simulink model "BugE_v0_40_MAS_loads"  (R2015b)
settings: Solver=FixedStepDiscrete  StartTime=0.0  StopTime=1980  FixedStep=sample_time  RelTol=1e-3
values from neighbouring files (symbols this model uses):
  AB_diode_dV = 0.9    [main_sync.m]
  air_density = 1.225    [main_sync.m]
  bus_charger_Pmax = 1000    [main_sync.m]
  bus_load_Pmax_abs = 250    [main_sync.m]
  capInitVolt = capVmax*sqrt(capInitSoC)    [main_sync.m]
  cyc_kph = [cyc_kph(:,1), cyc_kph(:,2)*speed_max_limit/speed_max]    [main_sync.m]
  cyc_repeat = 1    [main_sync.m]
  ess1_init_soc = 1    [main_sync.m]
  ess1_soh = 1    [main_sync.m]
  ess2_init_soc = 1    [main_sync.m]
  ess2_soh = 1    [main_sync.m]
  ess3_init_soc = 0.5    [main_sync.m]
  ess3_soh = 1    [main_sync.m]
  ess4_init_soc = 0.5    [main_sync.m]
  ess4_soh = 1    [main_sync.m]
  ess5_init_soc = 1    [main_sync.m]
  ess5_soh = 1    [main_sync.m]
  gear_ratio = 6    [main_sync.m]
  JADE_on = 1    [main_sync.m]
  loadpower = rawcsv(:,2)    [main_sync.m]
  loadtime = rawcsv(:,1)    [main_sync.m]
  lockSOCs = 0    [main_sync.m]
  max_brk_torque = 300    [main_sync.m]
  no_wheels = 3    [main_sync.m]
  period2 = max(loadtime)    [main_sync.m]
  PV_Pmax = 100    [main_sync.m]
  sample_time = 0.01    [main_sync.m]
  startup_seq_step_delay = 0.2    [main_sync.m]
  stop_option = 0    [main_sync.m]
  use_drive_cycle = 1    [main_sync.m]
  use_real_subs_loads = 1    [main_sync.m]
  vbus_max = 25    [main_sync.m]
  vbus_min = 17    [main_sync.m]
  vbus_safety_threshold = 2    [main_sync.m]
  vbus_threshold = 20    [main_sync.m]
  veh_CD = 0.35    [main_sync.m]
  veh_FA = 1.543    [main_sync.m]
  veh_gravity = 9.81*veh_mass    (= 1863.9)    [main_sync.m]
  veh_mass = 190    [main_sync.m]
  wh_1st_rrc = 0.02    [main_sync.m]
  wh_bearing_frc = 0.0015    [main_sync.m]
  wh_inertia = 0.0556    [main_sync.m]
  wh_radius = 0.508/2    (= 0.254)    [main_sync.m]
undefined symbols (not defined in the file or in its folder): capC, capR, cyc_acc, cyc_avg_time_samples, cyc_brk, cyc_grade, cyc_key, DCM_eff_factor_for_Vin, DCM_eff_for_Iout, DCM_Iout, DCM_Iout_max, DCM_Pin_noload, DCM_Pout_max, DCM_Vin, DCM_Vout, DiscIntNeverNeededParam, ess2_coulombic_eff, ess2_Ineg_max_SOC, ess2_Ineg_max_temp, ess2_Ipos_max_SOC, ess2_Ipos_max_temp, ess2_max_ah_cap, ess2_max_volts, ess2_min_volts, ess2_module_parallel, ess2_module_series, ess2_r_dis, ess2_soc, ess2_SOC_for_Ilimit, ess2_temp_for_Ilimit, ess2_temp_max, ess2_tmp, ess2_voc, ess3_coulombic_eff, ess3_max_ah_cap, ess3_module_parallel, ess3_module_series, ess3_r_dis, ess3_soc, ess3_tmp, ess3_voc, ess_coulombic_eff, ess_Ineg_max_SOC, ess_Ineg_max_temp, ess_Ipos_max_SOC, ess_Ipos_max_temp, ess_max_ah_cap, ess_max_volts, ess_min_volts, ess_module_parallel, ess_module_series, ess_nominal_volts, ess_r_dis, ess_soc, ess_SOC_for_Ilimit, ess_temp_for_Ilimit, ess_temp_max, ess_tmp, ess_voc, MC_eff1 ... (+17)
libraries: simulink x139, commfilt2 x1, simulink_extras x1
(part 1 of 7)
settings Model: Creator=gbucsan  LastModifiedBy=kcchu
settings DataIOCC: SaveFormat=Array
settings DebuggingCC: SolverPrmCheckMsg=warning  ParameterOverflowMsg=warning  AllowSymbolicDim=on
settings HardwareCC: ProdBitPerPointer=32  ProdLargestAtomicFloat=None  ProdIntDivRoundTo=Undefined  ProdEndianess=Unspecified  ProdWordSize=32  ProdHWDeviceType=32-bit Generic
settings ModelReferenceCC: ModelReferenceMinAlgLoopOccurrences=on
settings GRTTargetCC: GeneratePreprocessorConditionals=Disable all
settings ConfigComp: CovModelRefEnable=Off  CovSFcnEnable=off

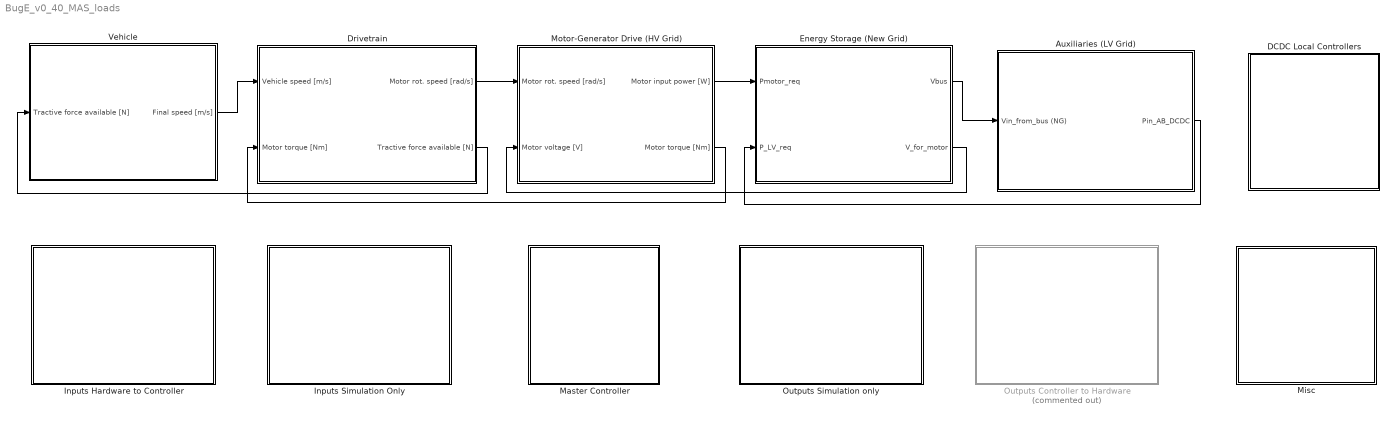
== system BugE_v0_40_MAS_loads ==
  Auxiliaries (LV Grid) : Subsystem
      mask Display: image('data\images\aux_systems2.png')
  DCDC Local Controllers : Subsystem
      mask Display: image('data\images\controller.png')
  Drivetrain : Subsystem
      mask Display: image('data\images\chain.jpg')
  Energy Storage (New Grid) : Subsystem
      mask Display: image('data\images\ess2.png')
  Inputs Hardware to Controller : Subsystem
      mask Display: image('data\images\in.png')
  Inputs Simulation Only : Subsystem
      mask Display: image('data\images\in.png')
  Master Controller : Subsystem
      mask Display: image('data\images\controller.png')
  Misc : Subsystem
      mask Display: image('data\images\debugger.png')
  Motor-Generator Drive (HV Grid) : Subsystem
      mask Display: image('data\images\motor.jpg')
  Outputs Controller to Hardware : Subsystem  Commented=on
      mask Display: image('data\images\out.png')
  Outputs Simulation only : Subsystem
      mask Display: image('data\images\out.png')
  Vehicle : Subsystem
      mask Display: image('data\images\bugev.png')
  wires:
  Vehicle/1(Final speed [m/s]) -> Drivetrain/1(Vehicle speed [m/s])
  Drivetrain/1(Motor rot. speed [rad/s]) -> Motor-Generator Drive (HV Grid)/1(Motor rot. speed [rad/s])
  Drivetrain/2(Tractive force available [N]) -> Vehicle/1(Tractive force available [N])
  Motor-Generator Drive (HV Grid)/2(Motor torque [Nm]) -> Drivetrain/2(Motor torque [Nm])
  Motor-Generator Drive (HV Grid)/1(Motor input power [W]) -> Energy Storage (New Grid)/1(Pmotor_req)
  Energy Storage (New Grid)/1("Vbus ") -> Auxiliaries (LV Grid)/1(Vin_from_bus (NG))
  Energy Storage (New Grid)/2(V_for_motor) -> Motor-Generator Drive (HV Grid)/2(Motor voltage [V])
  Auxiliaries (LV Grid)/1(Pin_AB_DCDC) -> Energy Storage (New Grid)/2(P_LV_req)

== system BugE_v0_40_MAS_loads/Auxiliaries (LV Grid) ==
  Vin_from_bus (NG) : Inport
  AB (w/ diode) : Subsystem
      mask Display: image('data\images\battery.jpg')
  AB DCDC : Subsystem
      mask Display: image('data\images\dcm.png')
  Auxiliary load (USB ports) : Subsystem
      mask Display: image('data\images\usb.jpg')
  Auxiliary load (lights) : Subsystem
      mask Display: image('data\images\auxiliaries.jpg')
  Constant : Constant  Value=0  SampleTime=sample_time
  ECU & sensors load : Subsystem
      mask Display: image('data\images\controller.png')
  P required on LV bus : Sum  Inputs=+++
  Switch1 : Switch  Criteria=u2 > Threshold
  Unit Delay1 : UnitDelay  InitialCondition=DCM_Pin_noload  SampleTime=sample_time
  Pin_AB_DCDC : Outport
  wires:
  Vin_from_bus (NG)/1 -> AB DCDC/1(Vin)
  AB DCDC/1(Pin_AB_DCDC (from new grid)) -> Unit Delay1/1
  Auxiliary load (lights)/1(power) -> P required on LV bus/1
  ECU & sensors load/1(power) -> P required on LV bus/2
  P required on LV bus/1 -> Switch1/1, AB DCDC/3(P_aux_req)
  [DDC] -> Switch1/2, AB DCDC/2(DCDC_enable)
  Switch1/1 -> AB (w/ diode)/1(Requested power [W])
  Unit Delay1/1 -> Pin_AB_DCDC/1
  Auxiliary load (USB ports)/1(power) -> P required on LV bus/3
  Constant/1 -> Switch1/3

== system BugE_v0_40_MAS_loads/DCDC Local Controllers ==
  Constant1 : Constant  Value=0
  Mux : Mux  Inputs=3
  Mux1 : Mux  Commented=on  Inputs=2
  Mux2 : Mux  Commented=on  Inputs=2
  Rate Transition3 : RateTransition
  Saturation Dynamic{,1..3} (4 alike) : simulink/Discontinuities/Saturation Dynamic  OutMin=[]  OutMax=[]  OutDataTypeStr=Inherit: Same as second input  OutDataType=fixdt(1, 16)  OutScaling=2^-10  DoSatur=off
  Scope : Scope  NumInputPorts=3
  To Workspace1 : ToWorkspace  VariableName=simout_Pmax_LD  SampleTime=1
  Unit Delay{1..4} (4 alike) : UnitDelay  SampleTime=-1
  flip sign : Gain  Gain=-1
  tag scope: PV_power_lim=global, ac_load_lim=global, autopilot_load_lim=global, charger_power_lim=global
  wires:
  [PV_power] -> Mux2/2, Saturation Dynamic/2  "pv"
  Constant1/1 -> Saturation Dynamic/3, Saturation Dynamic1/3, Saturation Dynamic3/3, Saturation Dynamic2/3
  [charger_power] -> Mux1/2, Saturation Dynamic1/2  "chg"
  [Chg_DCDC_command_value] -> Mux1/1, Saturation Dynamic1/1  "chg max"
  [Load_DCDC_command_value] -> flip sign/1  "load"
  flip sign/1 -> Rate Transition3/1, Mux/1, Saturation Dynamic3/1, Saturation Dynamic2/1  "load max"
  [autopilot_load] -> Mux/2, Saturation Dynamic2/2  "autopilot"
  Saturation Dynamic/1 -> Unit Delay1/1
  Saturation Dynamic1/1 -> Unit Delay2/1
  Saturation Dynamic2/1 -> Unit Delay3/1
  Unit Delay1/1 -> [PV_power_lim]
  Unit Delay2/1 -> [charger_power_lim]
  Unit Delay3/1 -> [autopilot_load_lim]
  [PV_DCDC_command_value] -> Mux2/1, Saturation Dynamic/1  "Pv max"
  Mux2/1 -> Scope/1
  Mux1/1 -> Scope/2
  Mux/1 -> Scope/3
  Saturation Dynamic3/1 -> Unit Delay4/1
  Unit Delay4/1 -> [ac_load_lim]
  [ac_load] -> Mux/3, Saturation Dynamic3/2  "A/C"
  Rate Transition3/1 -> To Workspace1/1

== system BugE_v0_40_MAS_loads/Drivetrain ==
  Vehicle speed [m/s] : Inport
  Motor torque [Nm] : Inport  Port=2
  "Brake_torque [Nm, abs]" : Gain  Gain=max_brk_torque
  Derivative : simulink/Discrete/Discrete Derivative  gainval=1.0  ICPrevScaledInput=0.0  InputProcessing=Inherited  OutMin=[]  OutMax=[]  OutDataType=fixdt(1, 16)  OutScaling=2^-10  DoSatur=off
  Energy Quantification : Subsystem
  Friction torque [Nm] : Product  Inputs=**
  Inertia torque [Nm] : Product  Inputs=**
  Speed [rad/s] : Product  Inputs=**
  Torque available at the wheel : Sum  Inputs=+---
  Torque available at the wheel sprocket from the motor [Nm] : Product
  Tractive force available : Product  Inputs=*/
  Wheel avg. rot. speed [rad/s] : Product  Inputs=/*
  "Wheel mom. of inertia [kg*m^2] " : Constant  Value=no_wheels*wh_inertia  SampleTime=sample_time
  gear ratio : Constant  Value=gear_ratio  SampleTime=sample_time
  wheel bearing viscous friction coeff.[Nm/(rad/s)] : Constant  Value=no_wheels*wh_bearing_frc  SampleTime=sample_time
  wheel radius [m] : Constant  Value=wh_radius  SampleTime=sample_time
  Motor rot. speed [rad/s] : Outport
  Tractive force available [N] : Outport  Port=2
  wires:
  Derivative/1 -> Inertia torque [Nm]/1
  wheel radius [m]/1 -> Tractive force available/2, Wheel avg. rot. speed [rad/s]/1
  Motor torque [Nm]/1 -> Torque available at the wheel sprocket from the motor [Nm]/2
  "Wheel mom. of inertia [kg*m^2] "/1 -> Inertia torque [Nm]/2
  wheel bearing viscous friction coeff.[Nm/(rad/s)]/1 -> Friction torque [Nm]/2
  Torque available at the wheel sprocket from the motor [Nm]/1 -> Torque available at the wheel/1
  Speed [rad/s]/1 -> Motor rot. speed [rad/s]/1
  Vehicle speed [m/s]/1 -> Wheel avg. rot. speed [rad/s]/2
  Tractive force available/1 -> Tractive force available [N]/1
  Torque available at the wheel/1 -> Tractive force available/1
  gear ratio/1 -> Speed [rad/s]/1, Torque available at the wheel sprocket from the motor [Nm]/1
  Inertia torque [Nm]/1 -> Torque available at the wheel/3, Energy Quantification/4(In4)
  Friction torque [Nm]/1 -> Energy Quantification/3(In3), Torque available at the wheel/2
  Wheel avg. rot. speed [rad/s]/1 -> Derivative/1, Friction torque [Nm]/1, Energy Quantification/2(In2), Speed [rad/s]/2
  "Brake_torque [Nm, abs]"/1 -> Energy Quantification/1(In1), Torque available at the wheel/4
  [brake] -> "Brake_torque [Nm, abs]"/1

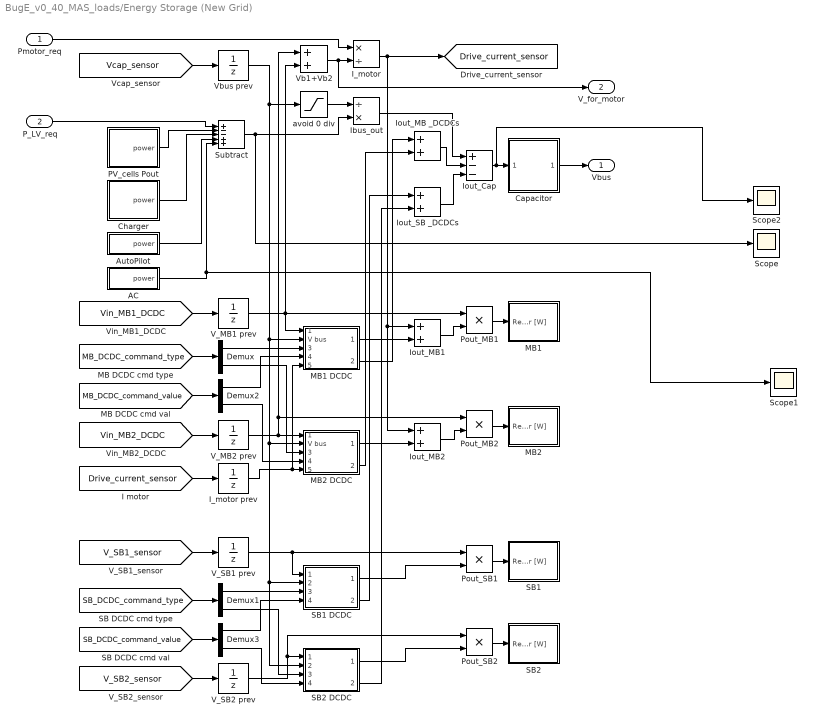
== system BugE_v0_40_MAS_loads/Energy Storage (New Grid) ==
  Pmotor_req : Inport
  P_LV_req : Inport  Port=2
  AC : Subsystem
  AutoPilot : Subsystem
  Capacitor : Subsystem
      mask Display: image('data\images\dlcap.jpg')
  Charger : Subsystem
      mask Display: image('data\images\v2g.jpg')
  Demux{,1..3} (4 alike) : Demux  Outputs=2
  I_motor : Product  Inputs=*/
  I_motor prev : UnitDelay  SampleTime=sample_time
  Ibus_out : Product  Inputs=/*
  Iout_Cap : Sum  Inputs=+--
  Iout_MB _DCDCs : Sum
  Iout_MB1 : Sum
  Iout_MB2 : Sum
  Iout_SB _DCDCs : Sum
  MB1 : Subsystem
      mask Display: image('data\images\battery.jpg')
  MB1 DCDC : Subsystem
      mask Display: image('data\images\dab.jpg')
  MB2 : Subsystem
      mask Display: image('data\images\battery.jpg')
  MB2 DCDC : Subsystem
      mask Display: image('data\images\dab.jpg')
  PV_cells Pout : Subsystem
      mask Display: image('data\images\pv.jpg')
  Pout_MB1 : Product
  Pout_MB2 : Product
  Pout_SB1 : Product
  Pout_SB2 : Product
  SB1 : Subsystem
      mask Display: image('data\images\battery.jpg')
  SB1 DCDC : Subsystem
      mask Display: image('data\images\dab.jpg')
  SB2 : Subsystem
      mask Display: image('data\images\battery.jpg')
  SB2 DCDC : Subsystem
      mask Display: image('data\images\dab.jpg')
  Scope : Scope
  Scope1 : Scope
  Scope2 : Scope
  Subtract : Sum  Inputs=+--++
  V_MB1 prev : UnitDelay  InitialCondition=ess_module_series*ess_max_volts  SampleTime=-1
  V_MB2 prev : UnitDelay  InitialCondition=ess_module_series*ess_max_volts  SampleTime=-1
  V_SB1 prev : UnitDelay  InitialCondition=ess2_module_series*ess2_max_volts  SampleTime=-1
  V_SB2 prev : UnitDelay  InitialCondition=ess2_module_series*ess2_max_volts  SampleTime=-1
  Vb1+Vb2 : Sum
  Vbus prev : UnitDelay  InitialCondition=capInitVolt  SampleTime=-1
  avoid 0 div : Saturate  UpperLimit=inf  LowerLimit=eps
  "Vbus " : Outport
  V_for_motor : Outport  Port=2
  tag scope: Drive_current_sensor=global
  wires:
  Pmotor_req/1 -> I_motor/1
  Vb1+Vb2/1 -> V_for_motor/1, I_motor/2
  MB1 DCDC/1(DAB_I_in) -> Iout_MB1/2
  MB2 DCDC/1(DAB_I_in) -> Iout_MB2/2
  Iout_MB2/1 -> Pout_MB2/2
  Iout_MB1/1 -> Pout_MB1/2
  Pout_MB1/1 -> MB1/1(Requested power [W])
  Pout_MB2/1 -> MB2/1(Requested power [W])
  MB2 DCDC/2(DAB_I_out) -> Iout_MB _DCDCs/2
  Ibus_out/1 -> Iout_Cap/1
  Subtract/1 -> Scope/1, Ibus_out/2
  Capacitor/1(Vbus) -> "Vbus "/1
  [Vin_MB1_DCDC] -> V_MB1 prev/1
  V_MB1 prev/1 -> MB1 DCDC/1(V batt), Vb1+Vb2/2, Pout_MB1/1
  [Vin_MB2_DCDC] -> V_MB2 prev/1
  V_MB2 prev/1 -> MB2 DCDC/1(V batt), Vb1+Vb2/1, Pout_MB2/1
  [Vcap_sensor] -> Vbus prev/1
  Iout_MB _DCDCs/1 -> Iout_Cap/2
  [V_SB1_sensor] -> V_SB1 prev/1
  V_SB1 prev/1 -> SB1 DCDC/1(V batt), Pout_SB1/1
  Vbus prev/1 -> MB2 DCDC/2(V bus), SB2 DCDC/2(V bus), SB1 DCDC/2(V bus), MB1 DCDC/2(V bus), avoid 0 div/1
  [V_SB2_sensor] -> V_SB2 prev/1
  V_SB2 prev/1 -> SB2 DCDC/1(V batt), Pout_SB2/1
  SB1 DCDC/1(DAB_I_in) -> Pout_SB1/2
  SB2 DCDC/1(DAB_I_in) -> Pout_SB2/2
  Pout_SB1/1 -> SB1/1(Requested power [W])
  Pout_SB2/1 -> SB2/1(Requested power [W])
  SB2 DCDC/2(DAB_I_out) -> Iout_SB _DCDCs/2
  SB1 DCDC/2(DAB_I_out) -> Iout_SB _DCDCs/1
  Iout_SB _DCDCs/1 -> Iout_Cap/3
  P_LV_req/1 -> Subtract/1
  PV_cells Pout/1(power) -> Subtract/2
  Charger/1(power) -> Subtract/3
  AutoPilot/1(power) -> Subtract/4
  avoid 0 div/1 -> Ibus_out/1
  Demux/1 -> MB1 DCDC/3("cmd type 0 P, 1 V ")
  [MB_DCDC_command_type] -> Demux/1
  [MB_DCDC_command_value] -> Demux2/1
  Demux2/1 -> MB1 DCDC/4(cmd value)
  [Drive_current_sensor] -> I_motor prev/1
  Demux/2 -> MB2 DCDC/3("cmd type 0 P, 1 V ")
  Demux2/2 -> MB2 DCDC/4(cmd value)
  I_motor prev/1 -> MB2 DCDC/5(I motor), MB1 DCDC/5(I motor)
  [SB_DCDC_command_type] -> Demux1/1
  [SB_DCDC_command_value] -> Demux3/1
  Demux1/1 -> SB1 DCDC/3("cmd type 0 P, 1 V ")
  Demux1/2 -> SB2 DCDC/3("cmd type 0 P, 1 V ")
  Demux3/1 -> SB1 DCDC/4(cmd value)
  Demux3/2 -> SB2 DCDC/4(cmd value)
  MB1 DCDC/2(DAB_I_out) -> Iout_MB _DCDCs/1
  I_motor/1 -> [Drive_current_sensor], Iout_MB1/1, Iout_MB2/1
  AC/1(power) -> Subtract/5, Scope1/1
  Iout_Cap/1 -> Scope2/1, Capacitor/1(Iout_RC)

== system BugE_v0_40_MAS_loads/Inputs Hardware to Controller ==
  Device detection & identification : Subsystem
  Sensors and readings : Subsystem
  User Inputs : Subsystem

== system BugE_v0_40_MAS_loads/Inputs Simulation Only ==
  AC load : Subsystem
  Autopilot load : Subsystem
  Auxiliaries power : Subsystem
  Charger power : Subsystem
  Clock1 : Clock
  Command Cycles : Subsystem
      mask Display: image('data\images\commands.png')
  PV power : Subsystem
  Standby load : Subsystem
  USB power : Subsystem
  dt : Constant  Value=sample_time  SampleTime=sample_time
  ess1_init_soc : Constant  Value=ess1_init_soc  SampleTime=sample_time
  ess2_init_soc : Constant  Value=ess2_init_soc  SampleTime=sample_time
  ess5_init_soc : Constant  Value=ess5_init_soc  SampleTime=sample_time
  repeat1 : Constant  Value=cyc_repeat  SampleTime=sample_time
  zero : Constant  Value=0  SampleTime=sample_time
  tag scope: AB_SOCinit=global, MB1_SOCinit=global, MB1_lower_SOH=global, MB2_SOCinit=global, PV_power=global, USB_load=global, ac_load=global, autopilot_load=global, aux_load=global, brake=global, charger_power=global, dt=global, endcycle_stopsim=global, grade=global, standby_load=global
  wires:
  zero/1 -> [MB1_lower_SOH]
  Standby load/1(Out1) -> [standby_load]
  Auxiliaries power/1(Out1) -> [aux_load]
  Autopilot load/1(Out1) -> [autopilot_load]
  Charger power/1(Out1) -> [charger_power]
  PV power/1(Out1) -> [PV_power]
  ess1_init_soc/1 -> [MB1_SOCinit]
  ess2_init_soc/1 -> [MB2_SOCinit]
  ess5_init_soc/1 -> [AB_SOCinit]
  Clock1/1 -> Command Cycles/2(Time)
  repeat1/1 -> Command Cycles/1(repeat)
  Command Cycles/2(endcycle_stopsim) -> [endcycle_stopsim]
  Command Cycles/3(grade) -> [grade]
  dt/1 -> [dt]
  Command Cycles/1(acc_brk_out) -> [brake]
  USB power/1(Out1) -> [USB_load]
  AC load/1(Out1) -> [ac_load]

== system BugE_v0_40_MAS_loads/Master Controller ==
  DCDC Calculators : Subsystem
  Detection : Subsystem
  Motor Controller : Subsystem
  Operating Mode Controller : Subsystem
  Secondary Objectives : Subsystem
  Signal Buffer : Subsystem
  System Health : Subsystem

== system BugE_v0_40_MAS_loads/Misc ==
  Data logging : Subsystem
  Debugging : Subsystem
  Energy Calculations : Subsystem
      mask Display: image('data\images\pie.png')
  STOP Sim : Subsystem

== system BugE_v0_40_MAS_loads/Motor-Generator Drive (HV Grid) ==
  Motor rot. speed [rad/s] : Inport
  Motor voltage [V] : Inport  Port=2
  Constant : Constant  Value=0  SampleTime=sample_time
  Current limiter : Subsystem
  Delay : Delay  DelayLength=1  SampleTime=sample_time
  Discrete Derivative : simulink/Discrete/Discrete Derivative  gainval=1.0  ICPrevScaledInput=0.0  InputProcessing=Inherited  OutMin=[]  OutMax=[]  OutDataType=fixdt(1, 16)  OutScaling=2^-10  DoSatur=off
  Efficiency map : Lookup_n-D  BreakpointsForDimension1=mc_map_spd*mc_spd_scale  BreakpointsForDimension2=mc_map_trq*mc_trq_scale  Table=mc_inpwr_map*mc_spd_scale*mc_trq_scale  InternalRulePriority=Speed  SaturateOnIntegerOverflow=on  InputSameDT=on
  Energy Quantification : Subsystem
  Gain : Gain  Gain=-1
  Inertia trq : Gain  Gain=mc_inertia
  Switch_Motor on/off : Switch  Criteria=u2 > Threshold
  Switch_Motor on/off1 : Switch  Criteria=u2 > Threshold
  Torque limiter : Subsystem
  Total torque output [Nm] : Sum  Inputs=+-
  Unit Delay prevent timing errors : UnitDelay  SampleTime=sample_time
  Motor input power [W] : Outport
  Motor torque [Nm] : Outport  Port=2
  wires:
  Efficiency map/1 -> Current limiter/1(Input power [W])
  Switch_Motor on/off/1 -> Energy Quantification/1(Pin), Motor input power [W]/1
  Torque limiter/1(Limited req. trq) -> Current limiter/3(Req. torque), Efficiency map/2
  Inertia trq/1 -> Energy Quantification/4(inertia torque), Gain/1, Total torque output [Nm]/2, Torque limiter/2(Inertia torque [Nm])
  Discrete Derivative/1 -> Inertia trq/1
  Motor voltage [V]/1 -> Current limiter/2(Voltage [V])
  Current limiter/1(Limited input power) -> Switch_Motor on/off/1
  Constant/1 -> Switch_Motor on/off/3
  [RLY_DRV] -> Unit Delay prevent timing errors/1
  Switch_Motor on/off1/1 -> Energy Quantification/3(torque out), Motor torque [Nm]/1
  Motor rot. speed [rad/s]/1 -> Discrete Derivative/1, Efficiency map/1, Energy Quantification/2(speed), Torque limiter/1(Speed [rad/s])
  Current limiter/2(Limited torque) -> Total torque output [Nm]/1
  Total torque output [Nm]/1 -> Switch_Motor on/off1/1
  Gain/1 -> Switch_Motor on/off1/3
  [throttle_adjusted] -> Delay/1
  Delay/1 -> Torque limiter/3(Requested throttle [0-1])
  Unit Delay prevent timing errors/1 -> Switch_Motor on/off/2, Switch_Motor on/off1/2

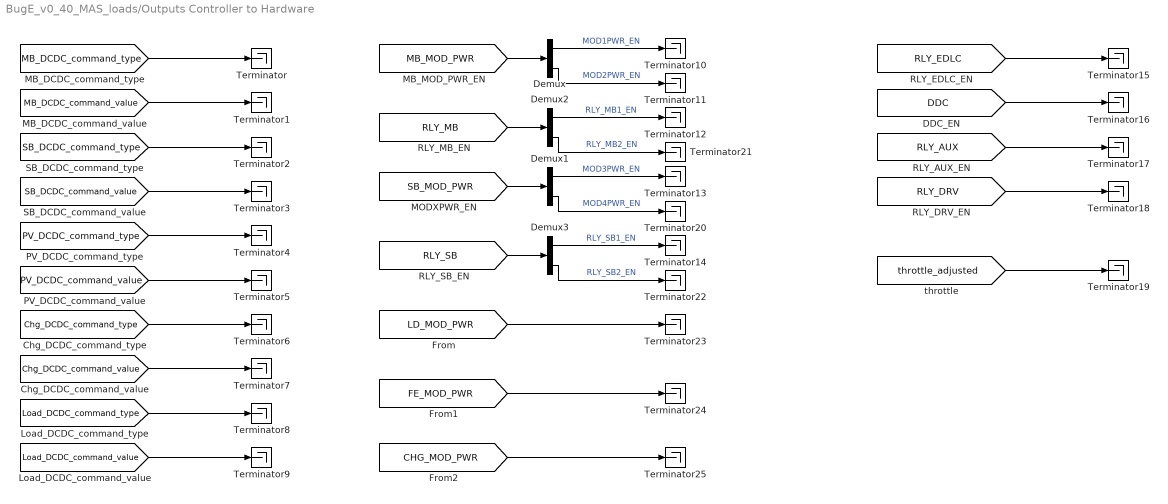
== system BugE_v0_40_MAS_loads/Outputs Controller to Hardware ==
  Demux{,1..3} (4 alike) : Demux  Outputs=2
  Terminator{,1..25} (26 alike) : Terminator
  wires:
  [MB_DCDC_command_type] -> Terminator/1
  [MB_DCDC_command_value] -> Terminator1/1
  [SB_DCDC_command_type] -> Terminator2/1
  [SB_DCDC_command_value] -> Terminator3/1
  [PV_DCDC_command_type] -> Terminator4/1
  [PV_DCDC_command_value] -> Terminator5/1
  [Chg_DCDC_command_type] -> Terminator6/1
  [Chg_DCDC_command_value] -> Terminator7/1
  [Load_DCDC_command_type] -> Terminator8/1
  [Load_DCDC_command_value] -> Terminator9/1
  Demux/1 -> Terminator10/1  "MOD1PWR_EN"
  Demux/2 -> Terminator11/1  "MOD2PWR_EN"
  [RLY_EDLC] -> Terminator15/1
  [DDC] -> Terminator16/1
  [RLY_AUX] -> Terminator17/1
  [RLY_DRV] -> Terminator18/1
  [throttle_adjusted] -> Terminator19/1
  [MB_MOD_PWR] -> Demux/1
  Demux1/1 -> Terminator13/1  "MOD3PWR_EN"
  Demux1/2 -> Terminator20/1  "MOD4PWR_EN"
  [SB_MOD_PWR] -> Demux1/1
  Demux2/1 -> Terminator12/1  "RLY_MB1_EN"
  Demux2/2 -> Terminator21/1  "RLY_MB2_EN"
  [RLY_MB] -> Demux2/1
  Demux3/1 -> Terminator14/1  "RLY_SB1_EN"
  Demux3/2 -> Terminator22/1  "RLY_SB2_EN"
  [RLY_SB] -> Demux3/1
  [LD_MOD_PWR] -> Terminator23/1
  [FE_MOD_PWR] -> Terminator24/1
  [CHG_MOD_PWR] -> Terminator25/1

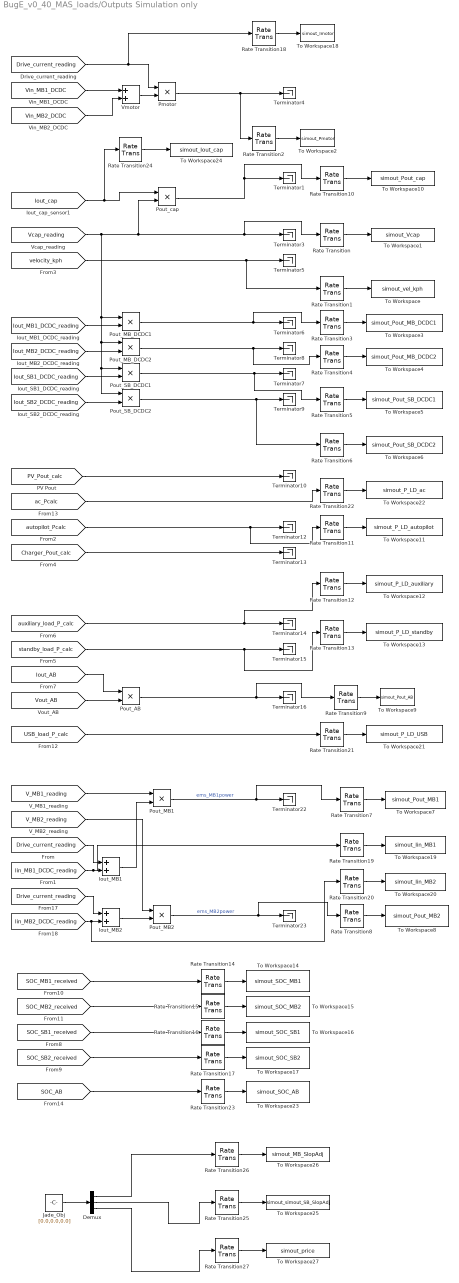
== system BugE_v0_40_MAS_loads/Outputs Simulation only ==
  Demux : Demux  Outputs=3
  Iout_MB1 : Sum
  Iout_MB2 : Sum
  Jade_Obj : Constant  Value=[0.0,0.0,0.0]  SampleTime=sample_time
  Pmotor : Product
  Pout_AB : Product
  Pout_MB1 : Product
  Pout_MB2 : Product
  Pout_MB_DCDC1 : Product
  Pout_MB_DCDC2 : Product
  Pout_SB_DCDC1 : Product
  Pout_SB_DCDC2 : Product
  Pout_cap : Product
  Rate Transition{,1..27} (28 alike) : RateTransition
  Terminator{1,3..10,12..16,22..23} (16 alike) : Terminator
  To Workspace : ToWorkspace  VariableName=simout_vel_kph  SampleTime=1
  To Workspace1 : ToWorkspace  VariableName=simout_Vcap  SampleTime=1
      settings: MaxDataPoints=Inf
  To Workspace10 : ToWorkspace  VariableName=simout_Pout_cap  SampleTime=1
      settings: MaxDataPoints=Inf
  To Workspace11 : ToWorkspace  VariableName=simout_P_LD_autopilot  SampleTime=1
  To Workspace12 : ToWorkspace  VariableName=simout_P_LD_auxiliary  SampleTime=1
  To Workspace13 : ToWorkspace  VariableName=simout_P_LD_standby  SampleTime=1
  To Workspace14 : ToWorkspace  VariableName=simout_SOC_MB1  SampleTime=1
  To Workspace15 : ToWorkspace  VariableName=simout_SOC_MB2  SampleTime=1
  To Workspace16 : ToWorkspace  VariableName=simout_SOC_SB1  SampleTime=1
  To Workspace17 : ToWorkspace  VariableName=simout_SOC_SB2  SampleTime=1
  To Workspace18 : ToWorkspace  VariableName=simout_Imotor  SampleTime=1
  To Workspace19 : ToWorkspace  VariableName=simout_Iin_MB1  SampleTime=1
  To Workspace2 : ToWorkspace  VariableName=simout_Pmotor  SampleTime=1
  To Workspace20 : ToWorkspace  VariableName=simout_Iin_MB2  SampleTime=1
  To Workspace21 : ToWorkspace  VariableName=simout_P_LD_USB  SampleTime=1
  To Workspace22 : ToWorkspace  VariableName=simout_P_LD_ac  SampleTime=1
  To Workspace23 : ToWorkspace  VariableName=simout_SOC_AB  SampleTime=1
  To Workspace24 : ToWorkspace  VariableName=simout_Iout_cap  SampleTime=1
      settings: MaxDataPoints=Inf
  To Workspace25 : ToWorkspace  VariableName=simout_simout_SB_SlopAdj  SampleTime=1
      settings: MaxDataPoints=Inf
  To Workspace26 : ToWorkspace  VariableName=simout_MB_SlopAdj  SampleTime=1
      settings: MaxDataPoints=Inf
  To Workspace27 : ToWorkspace  VariableName=simout_price  SampleTime=1
      settings: MaxDataPoints=Inf
  To Workspace3 : ToWorkspace  VariableName=simout_Pout_MB_DCDC1  SampleTime=1
  To Workspace4 : ToWorkspace  VariableName=simout_Pout_MB_DCDC2  SampleTime=1
  To Workspace5 : ToWorkspace  VariableName=simout_Pout_SB_DCDC1  SampleTime=1
  To Workspace6 : ToWorkspace  VariableName=simout_Pout_SB_DCDC2  SampleTime=1
  To Workspace7 : ToWorkspace  VariableName=simout_Pout_MB1  SampleTime=1
  To Workspace8 : ToWorkspace  VariableName=simout_Pout_MB2  SampleTime=1
  To Workspace9 : ToWorkspace  VariableName=simout_Pout_AB  SampleTime=1
  Vmotor : Sum
  wires:
  Vmotor/1 -> Pmotor/2
  [Vin_MB2_DCDC] -> Vmotor/2
  [Drive_current_reading] -> Rate Transition18/1, Pmotor/1
  Pmotor/1 -> Rate Transition2/1, Terminator4/1
  [Vin_MB1_DCDC] -> Vmotor/1
  [Vcap_reading] -> Pout_cap/2, Rate Transition/1, Terminator3/1, Pout_SB_DCDC2/1, Pout_SB_DCDC1/1, Pout_MB_DCDC2/1, Pout_MB_DCDC1/1
  [velocity_kph] -> Rate Transition1/1, Terminator5/1
  [Iout_MB1_DCDC_reading] -> Pout_MB_DCDC1/2
  [Iout_MB2_DCDC_reading] -> Pout_MB_DCDC2/2
  [Iout_SB1_DCDC_reading] -> Pout_SB_DCDC1/2
  [Iout_SB2_DCDC_reading] -> Pout_SB_DCDC2/2
  Pout_MB_DCDC1/1 -> Rate Transition3/1, Terminator6/1
  Pout_MB_DCDC2/1 -> Rate Transition4/1, Terminator8/1
  Pout_SB_DCDC1/1 -> Rate Transition5/1, Terminator7/1
  Pout_SB_DCDC2/1 -> Rate Transition6/1, Terminator9/1
  [PV_Pout_calc] -> Terminator10/1
  [autopilot_Pcalc] -> Rate Transition11/1, Terminator12/1
  [Charger_Pout_calc] -> Terminator13/1
  [Vout_AB] -> Pout_AB/2
  [Iout_AB] -> Pout_AB/1
  Pout_AB/1 -> Rate Transition9/1, Terminator16/1
  Iout_MB2/1 -> Pout_MB2/2
  [V_MB2_reading] -> Pout_MB2/1
  [V_MB1_reading] -> Pout_MB1/1
  Iout_MB1/1 -> Pout_MB1/2
  Pout_MB1/1 -> Rate Transition7/1, Terminator22/1  "ems_MB1power"
  Pout_MB2/1 -> Rate Transition8/1, Terminator23/1  "ems_MB2power"
  [Drive_current_reading] -> Iout_MB1/1
  [Iin_MB1_DCDC_reading] -> Rate Transition19/1, Iout_MB1/2
  [Drive_current_reading] -> Iout_MB2/1
  [Iin_MB2_DCDC_reading] -> Rate Transition20/1, Iout_MB2/2
  Rate Transition/1 -> To Workspace1/1
  Rate Transition1/1 -> To Workspace/1
  Rate Transition2/1 -> To Workspace2/1
  Rate Transition3/1 -> To Workspace3/1
  Rate Transition4/1 -> To Workspace4/1
  Rate Transition5/1 -> To Workspace5/1
  Rate Transition6/1 -> To Workspace6/1
  Rate Transition7/1 -> To Workspace7/1
  Rate Transition8/1 -> To Workspace8/1
  Rate Transition9/1 -> To Workspace9/1
  [Iout_cap] -> Rate Transition24/1, Pout_cap/1
  Pout_cap/1 -> Rate Transition10/1, Terminator1/1
  Rate Transition10/1 -> To Workspace10/1
  Rate Transition11/1 -> To Workspace11/1
  [auxiliary_load_P_calc] -> Rate Transition12/1, Terminator14/1
  Rate Transition12/1 -> To Workspace12/1
  [standby_load_P_calc] -> Rate Transition13/1, Terminator15/1
  Rate Transition13/1 -> To Workspace13/1
  Rate Transition14/1 -> To Workspace14/1
  [SOC_MB1_received] -> Rate Transition14/1
  Rate Transition15/1 -> To Workspace15/1
  [SOC_MB2_received] -> Rate Transition15/1
  Rate Transition16/1 -> To Workspace16/1
  [SOC_SB1_received] -> Rate Transition16/1
  Rate Transition17/1 -> To Workspace17/1
  [SOC_SB2_received] -> Rate Transition17/1
  Rate Transition18/1 -> To Workspace18/1
  Rate Transition19/1 -> To Workspace19/1
  Rate Transition20/1 -> To Workspace20/1
  [USB_load_P_calc] -> Rate Transition21/1
  Rate Transition21/1 -> To Workspace21/1
  Rate Transition22/1 -> To Workspace22/1
  [ac_Pcalc] -> Rate Transition22/1
  Rate Transition23/1 -> To Workspace23/1
  [SOC_AB] -> Rate Transition23/1
  Rate Transition24/1 -> To Workspace24/1
  Jade_Obj/1 -> Demux/1
  Demux/2 -> Rate Transition25/1
  Rate Transition25/1 -> To Workspace25/1
  Demux/1 -> Rate Transition26/1
  Rate Transition26/1 -> To Workspace26/1
  Demux/3 -> Rate Transition27/1
  Rate Transition27/1 -> To Workspace27/1

== system BugE_v0_40_MAS_loads/Vehicle ==
  Tractive force available [N] : Inport
  Achievable vehicle speed : Subsystem
  Unit Delay : UnitDelay  SampleTime=-1
  "m/s -> km/h" : Gain  Gain=3.6
  Final speed [m/s] : Outport
  tag scope: velocity_kph=global
  wires:
  Tractive force available [N]/1 -> Achievable vehicle speed/2(Available avg. tractive force [N])
  Achievable vehicle speed/1(Vehicle speed at the end of time step [m/s]) -> Unit Delay/1, "m/s -> km/h"/1
  "m/s -> km/h"/1 -> [velocity_kph]
  Unit Delay/1 -> Achievable vehicle speed/1(Vehicle speed at the beginning of the time step [m/s]), Final speed [m/s]/1

== system BugE_v0_40_MAS_loads/Auxiliaries (LV Grid)/AB (w// diode) ==
  Requested power [W] : Inport
  AB_diode_dV : Constant  Value=AB_diode_dV  SampleTime=sample_time
  Calculate SOC : Subsystem
  Compute current (nolimit) : Subsystem
  Constant : Constant  Value=25  SampleTime=sample_time
  Energy Quantification : Subsystem
  "Pack Voc, R" : Subsystem
  Scope : Scope
  tag scope: Iout_AB=global, SOC_AB=global, Vout_AB=global
  wires:
  Requested power [W]/1 -> "Pack Voc, R"/3(Req. power [W]), Compute current (nolimit)/3(Output power [W])
  "Pack Voc, R"/1(Pack Voc [V]) -> Compute current (nolimit)/1(Voc [V])
  Constant/1 -> Calculate SOC/1(Temp [C]), "Pack Voc, R"/1(Temp [degC])
  [SOC_AB] -> "Pack Voc, R"/2(SOC_prev)
  "Pack Voc, R"/2(Pack R [Ohm]) -> Energy Quantification/3(R), Compute current (nolimit)/2(Rint [Ohm])
  Compute current (nolimit)/1(I [A]) -> Calculate SOC/2(I [A]), [Iout_AB], Energy Quantification/2(Iout)
  AB_diode_dV/1 -> Compute current (nolimit)/4(diode_dV [V]), Energy Quantification/4(diode_dV [V])
  Compute current (nolimit)/2(V_out [V]) -> Energy Quantification/1(Vout), [Vout_AB]
  Calculate SOC/1(SOC) -> Scope/1, [SOC_AB]

== system BugE_v0_40_MAS_loads/Auxiliaries (LV Grid)/AB DCDC ==
  Vin : Inport
  DCDC_enable : Inport  Port=2
  P_aux_req : Inport  Port=3
  >0 avoid 0 div : Saturate  UpperLimit=inf  LowerLimit=eps
  Comp 0 : simulink/Logic and Bit Operations/Compare To Zero  relop===  OutDataTypeStr=boolean
  Constant : Constant  Value=0  SampleTime=sample_time
  DCM: Iout->eff : Lookup_n-D  NumberOfTableDimensions=1  BreakpointsForDimension1=DCM_Iout(:)  Table=DCM_eff_for_Iout(:)  InterpMethod=Cubic spline  ExtrapMethod=Clip  InternalRulePriority=Speed  RndMeth=Simplest  InputSameDT=on
  Energy Quantification : Subsystem
  Iin : Product  Inputs=*/
  Imax : Constant  Value=DCM_Iout_max  SampleTime=sample_time
  Iout : Product  Inputs=*/
  Iout_AB_DCDC_sensor : Goto  Commented=on  GotoTag=Iout_AB_DCDC_sensor  TagVisibility=global
  Min : MinMax  Inputs=2
  P=0 for shutdown : Switch  Criteria=u2 > Threshold
  P_noload : Constant  Value=DCM_Pin_noload  SampleTime=sample_time
  Pin_init : Product  Inputs=*/
  Pin_init1 : Product  Inputs=*/
  Pmax : MinMax  Inputs=2
  Pmax_calc : Product
  Pmax_given : Constant  Value=DCM_Pout_max*2  SampleTime=sample_time
  Pout : Product  Inputs=**
  Pout_AB_DCDC (into LV grid) : Switch  Criteria=u2 > Threshold
  Saturation : simulink/Discontinuities/Saturation Dynamic  OutMin=[]  OutMax=[]  OutDataTypeStr=Inherit: Same as second input  OutDataType=fixdt(1, 16)  OutScaling=2^-10  DoSatur=off
  Unit Delay : UnitDelay  InitialCondition=23  SampleTime=-1
  Vin->eff_factor : Lookup_n-D  NumberOfTableDimensions=1  BreakpointsForDimension1=DCM_Vin(:)  Table=DCM_eff_factor_for_Vin(:)  InterpMethod=Cubic spline  InternalRulePriority=Speed  RndMeth=Simplest  InputSameDT=on
  Vout = 12V : Constant  Value=DCM_Vout  SampleTime=sample_time
  disabled : Logic  Operator=NOT  AllPortsSameDT=off  OutDataTypeStr=boolean
  eff : Product  Inputs=**
  normal or no-load : Switch  Criteria=u2 > Threshold
  off or no-load : Logic  Operator=OR  AllPortsSameDT=off  OutDataTypeStr=boolean
  Pin_AB_DCDC (from new grid) : Outport
  tag scope: Iin_AB_DCDC_sensor=global
  wires:
  Vin->eff_factor/1 -> eff/2
  Vin/1 -> Unit Delay/1
  DCM: Iout->eff/1 -> eff/1
  P_aux_req/1 -> Pin_init/1, Iout/1
  eff/1 -> Pout/1, Pin_init/2
  Iout/1 -> DCM: Iout->eff/1
  Saturation/1 -> normal or no-load/3, Comp 0/1
  Comp 0/1 -> normal or no-load/2, off or no-load/2
  P_noload/1 -> normal or no-load/1
  P=0 for shutdown/1 -> Energy Quantification/2(In2), Iin/1, Pout/2, Pin_AB_DCDC (from new grid)/1
  Min/1 -> Pmax_calc/1
  Imax/1 -> Pmax_calc/2
  Pmax_calc/1 -> Pmax/1
  Pmax_given/1 -> Pmax/2
  Pmax/1 -> Saturation/1
  Pin_init/1 -> Saturation/2
  Pout_AB_DCDC (into LV grid)/1 -> Pin_init1/1, Energy Quantification/1(In1)
  Unit Delay/1 -> Vin->eff_factor/1, >0 avoid 0 div/1, Min/1
  Iin/1 -> [Iin_AB_DCDC_sensor]
  disabled/1 -> off or no-load/1, P=0 for shutdown/2
  Constant/1 -> Pout_AB_DCDC (into LV grid)/1, P=0 for shutdown/1, Saturation/3
  Pout/1 -> Pout_AB_DCDC (into LV grid)/3
  off or no-load/1 -> Pout_AB_DCDC (into LV grid)/2
  DCDC_enable/1 -> disabled/1
  normal or no-load/1 -> P=0 for shutdown/3
  Vout = 12V/1 -> Min/2, Iout/2, Pin_init1/2
  Pin_init1/1 -> Iout_AB_DCDC_sensor/1
  >0 avoid 0 div/1 -> Iin/2

== system BugE_v0_40_MAS_loads/Auxiliaries (LV Grid)/Auxiliary load (USB ports) ==
  Constant : Constant  Value=0  SampleTime=sample_time
  Constant1 : Constant  Value=JADE_on
  Demux : Demux  Outputs=3
  Energy Quantification : Subsystem
  Jade_LD_USB : Constant  Value=[0.0,0.0,0.0]  SampleTime=sample_time
  Pmax : Terminator
  Rate Transition24 : RateTransition
  Switch : Switch  Criteria=u2 > Threshold
  Switch2 : Switch  Criteria=u2 > Threshold
  To Workspace24 : ToWorkspace  VariableName=simout_Level_usb  SampleTime=1
      settings: MaxDataPoints=Inf
  USB level : Gain
  level : Terminator
  power : Outport
  tag scope: USB_load_P_calc=global
  wires:
  Constant/1 -> Switch/3
  [RLY_AUX] -> Switch/2
  Switch/1 -> USB level/1
  USB level/1 -> power/1, Energy Quantification/1(Power), [USB_load_P_calc]
  Constant1/1 -> Switch2/2
  Jade_LD_USB/1 -> Demux/1
  Demux/3 -> Switch2/1
  Demux/1 -> Pmax/1
  Switch2/1 -> Switch/1
  [USB_load] -> Switch2/3
  Demux/2 -> Rate Transition24/1, level/1
  Rate Transition24/1 -> To Workspace24/1

== system BugE_v0_40_MAS_loads/Auxiliaries (LV Grid)/Auxiliary load (lights) ==
  Constant : Constant  Value=0  SampleTime=sample_time
  Constant1 : Constant  Value=JADE_on
  Demux : Demux  Outputs=3
  Energy Quantification : Subsystem
  Jade_LD_Lights : Constant  Value=[0.0,0.0,0.0]  SampleTime=sample_time
  Pmax : Terminator
  Rate Transition24 : RateTransition
  Switch : Switch  Criteria=u2 > Threshold
  Switch2 : Switch  Criteria=u2 > Threshold
  To Workspace24 : ToWorkspace  VariableName=simout_Level_lights  SampleTime=1
      settings: MaxDataPoints=Inf
  level : Terminator
  power : Outport
  tag scope: auxiliary_load_P_calc=global
  wires:
  Constant/1 -> Switch/3
  [RLY_AUX] -> Switch/2
  Switch/1 -> power/1, Energy Quantification/1(Power), [auxiliary_load_P_calc]
  Constant1/1 -> Switch2/2
  Jade_LD_Lights/1 -> Demux/1
  Demux/3 -> Switch2/1
  Demux/2 -> Rate Transition24/1, level/1
  Demux/1 -> Pmax/1
  [aux_load] -> Switch2/3
  Switch2/1 -> Switch/1
  Rate Transition24/1 -> To Workspace24/1

== system BugE_v0_40_MAS_loads/Auxiliaries (LV Grid)/ECU & sensors load ==
  Energy Quantification : Subsystem
  power : Outport
  tag scope: standby_load_P_calc=global
  wires:
  [standby_load] -> power/1, [standby_load_P_calc], Energy Quantification/1(Power)

== system BugE_v0_40_MAS_loads/Drivetrain/Energy Quantification ==
  In1 : Inport
  In2 : Inport  Port=2
  In3 : Inport  Port=3
  In4 : Inport  Port=4
  > 0 : Saturate  UpperLimit=inf  LowerLimit=0
  Product : Product
  Product1 : Product
  Product2 : Product
  tag scope: E_mech_brake=global, E_wh_bearing=global, E_wh_inertia=global
  wires:
  Product/1 -> [E_wh_bearing]
  Product2/1 -> > 0/1
  Product1/1 -> [E_mech_brake]
  > 0/1 -> [E_wh_inertia]
  In2/1 -> Product/2, Product2/1, Product1/2
  In3/1 -> Product/1
  In1/1 -> Product1/1
  In4/1 -> Product2/2

== system BugE_v0_40_MAS_loads/Energy Storage (New Grid)/AC ==
  Constant : Constant  Value=JADE_on
  Demux : Demux  Outputs=3
  Energy Quantification : Subsystem
  Jade_LD_AC : Constant  Value=[0.0,0.0,0.0]  SampleTime=sample_time
  Pmax : Terminator
  Rate Transition24 : RateTransition
  Switch2 : Switch  Criteria=u2 > Threshold
  To Workspace24 : ToWorkspace  VariableName=simout_Level_ac  SampleTime=1
      settings: MaxDataPoints=Inf
  level : Terminator
  power : Outport
  tag scope: ac_Pcalc=global
  wires:
  Constant/1 -> Switch2/2
  Jade_LD_AC/1 -> Demux/1
  Demux/3 -> Switch2/1
  Demux/1 -> Pmax/1
  [ac_load_lim] -> Switch2/3
  Switch2/1 -> Energy Quantification/1(Power), power/1, [ac_Pcalc]
  Demux/2 -> Rate Transition24/1, level/1
  Rate Transition24/1 -> To Workspace24/1

== system BugE_v0_40_MAS_loads/Energy Storage (New Grid)/AutoPilot ==
  Constant : Constant  Value=JADE_on
  Demux : Demux  Outputs=3
  Energy Quantification : Subsystem
  Jade_LD_Autopilot : Constant  Value=[0.0,0.0,0.0]  SampleTime=sample_time
  Pmax : Terminator
  Rate Transition24 : RateTransition
  Switch2 : Switch  Criteria=u2 > Threshold
  To Workspace24 : ToWorkspace  VariableName=simout_Level_autopilot  SampleTime=1
      settings: MaxDataPoints=Inf
  level : Terminator
  power : Outport
  tag scope: autopilot_Pcalc=global
  wires:
  Constant/1 -> Switch2/2
  [autopilot_load_lim] -> Switch2/3
  Switch2/1 -> power/1, Energy Quantification/1(Power), [autopilot_Pcalc]
  Jade_LD_Autopilot/1 -> Demux/1
  Demux/3 -> Switch2/1
  Demux/1 -> Pmax/1
  Demux/2 -> Rate Transition24/1, level/1
  Rate Transition24/1 -> To Workspace24/1

== system BugE_v0_40_MAS_loads/Energy Storage (New Grid)/Capacitor ==
  Iout_RC : Inport
  Energy Quantification : Subsystem
  Iin : Gain  Gain=-1
  Switch : Switch  Criteria=u2 > Threshold
  Switch1 : Switch  Criteria=u2 > Threshold
  V_capRC : Sum
  Vcap : Gain  Gain=1/capC
  VcapR (<0) : Product
  cap Q : DiscreteIntegrator  InitialCondition=capC*capInitVolt  InitialConditionSetting=State (most efficient)  SampleTime=sample_time  ICPrevOutput=DiscIntNeverNeededParam  ICPrevScaledInput=DiscIntNeverNeededParam
  capR : Constant  Value=capR  SampleTime=sample_time
  prevent timing errors : UnitDelay  SampleTime=sample_time
  zero : Constant  Value=0  SampleTime=sample_time
  Vbus : Outport
  tag scope: Iout_cap=global, Vcap_sensor=global
  wires:
  cap Q/1 -> Vcap/1
  VcapR (<0)/1 -> V_capRC/1
  Switch/1 -> Energy Quantification/3(Iout), [Iout_cap], Iin/1
  Switch1/1 -> Energy Quantification/2(Vcap_RC), [Vcap_sensor], Vbus/1
  Iin/1 -> VcapR (<0)/2, cap Q/1
  capR/1 -> Energy Quantification/1(R), VcapR (<0)/1
  Vcap/1 -> V_capRC/2
  [RLY_EDLC] -> prevent timing errors/1
  Iout_RC/1 -> Switch/1
  zero/1 -> Switch1/3, Switch/3
  V_capRC/1 -> Switch1/1
  prevent timing errors/1 -> Switch1/2, Switch/2

== system BugE_v0_40_MAS_loads/Energy Storage (New Grid)/Charger ==
  Energy Quantification : Subsystem
  power : Outport
  tag scope: Charger_Pout_calc=global
  wires:
  [charger_power_lim] -> Energy Quantification/1(Power), power/1, [Charger_Pout_calc]

== system BugE_v0_40_MAS_loads/Energy Storage (New Grid)/MB1 ==
  Requested power [W] : Inport
  Calculate SOC : Subsystem
  Compute current (nolimit) : Subsystem
  Constant : Constant  Value=0  SampleTime=sample_time
  Demux : Demux  Outputs=2
  Energy Quantification : Subsystem
  "Pack Voc, R" : Subsystem
  Switch : Switch  Criteria=u2 > Threshold
  Terminator : Terminator
  and : Logic  AllPortsSameDT=off  OutDataTypeStr=boolean
  prevent timing errors : UnitDelay  SampleTime=sample_time
  tag scope: SOC_MB1=global, V_MB1_sensor=global
  wires:
  Switch/1 -> Compute current (nolimit)/3(Output power [W]), "Pack Voc, R"/2(Req. power [W])
  "Pack Voc, R"/1(Pack Voc [V]) -> Compute current (nolimit)/1(Voc [V])
  [temp_MB1_sensor] -> "Pack Voc, R"/3(Temp [degC]), Calculate SOC/1(Temp [C])
  [SOC_MB1] -> "Pack Voc, R"/1(SOC_prev)
  "Pack Voc, R"/2(Pack R [Ohm]) -> Energy Quantification/3(R), Compute current (nolimit)/2(Rint [Ohm])
  Compute current (nolimit)/1(I [A]) -> Energy Quantification/2(I), Calculate SOC/2(I [A])
  Compute current (nolimit)/2(V [V]) -> Energy Quantification/1(V), [V_MB1_sensor]
  Constant/1 -> Switch/3
  Requested power [W]/1 -> Switch/1
  Demux/1 -> Switch/2
  [RLY_MB] -> and/1
  Demux/2 -> Terminator/1
  prevent timing errors/1 -> Demux/1
  [MB_MOD_PWR] -> and/2
  and/1 -> prevent timing errors/1
  Calculate SOC/1(SOC) -> [SOC_MB1]

== system BugE_v0_40_MAS_loads/Energy Storage (New Grid)/MB1 DCDC ==
  V batt : Inport
  V bus : Inport  Port=2
  "cmd type 0 P, 1 V " : Inport  Port=3
  cmd value : Inport  Port=4
  I motor : Inport  Port=5
  0 : Constant  Value=eps  SampleTime=sample_time
  Current limiter : Subsystem
  Demux : Demux  Outputs=2
  Demux1 : Demux  Outputs=2
  Demux2 : Demux  Outputs=2
  Energy Quantification : Subsystem
  Imax abs : Constant  Value=MC_Imax  SampleTime=sample_time
  Scope : Scope  NumInputPorts=3
  Term : Terminator
  Term1 : Terminator
  V MB nominal : Constant  Value=ess_nominal_volts*ess_module_series  SampleTime=sample_time
  eff_maps : Subsystem
  eff_maps1 : Subsystem
  enabled : Switch  Criteria=u2 > Threshold
  failure mode (Voltage mode) : Switch  Criteria=u2 > Threshold
  prevent timing errors{,1..3} (4 alike) : UnitDelay  SampleTime=sample_time
  switch2 : Switch  Criteria=u2 > Threshold
  DAB_I_in : Outport
  DAB_I_out : Outport  Port=2
  tag scope: Iin_MB1_DCDC_sensor=global, Iout_MB1_DCDC_sensor=global, Vin_MB1_DCDC=global
  wires:
  Current limiter/2(I bus side lim) -> Scope/2, Energy Quantification/1(In1), DAB_I_out/1, [Iout_MB1_DCDC_sensor]
  Current limiter/1(I batt side lim) -> Scope/1, [Iin_MB1_DCDC_sensor], DAB_I_in/1, Energy Quantification/3(In3)
  V MB nominal/1 -> failure mode (Voltage mode)/3
  failure mode (Voltage mode)/1 -> enabled/1
  [RLY_MB] -> prevent timing errors3/1
  [V_MB1_sensor] -> failure mode (Voltage mode)/1
  Demux/1 -> failure mode (Voltage mode)/2
  Demux/2 -> Term/1
  Imax abs/1 -> Current limiter/4(I max)
  cmd value/1 -> prevent timing errors2/1
  V batt/1 -> eff_maps/3(Vbatt), Energy Quantification/4(In4)
  V bus/1 -> eff_maps/2(Vbus), Energy Quantification/2(In2), eff_maps1/3(Vbus)
  Demux1/1 -> Current limiter/2(I batt side raw)
  Demux1/2 -> Current limiter/3(I bus side raw)
  "cmd type 0 P, 1 V "/1 -> prevent timing errors1/1
  eff_maps/1(I from batt & into bus) -> switch2/3
  I motor/1 -> eff_maps1/1(I motor)
  switch2/1 -> Demux1/1
  [MB_MOD_PWR] -> prevent timing errors/1
  Demux2/2 -> Term1/1
  enabled/1 -> [Vin_MB1_DCDC]
  0/1 -> enabled/3
  Demux2/1 -> Current limiter/1(enable DCDC), enabled/2
  prevent timing errors/1 -> Demux2/1
  prevent timing errors1/1 -> switch2/2
  prevent timing errors3/1 -> Demux/1
  prevent timing errors2/1 -> eff_maps/1("P into bus cmd "), eff_maps1/2(Vbatt cmd)
  eff_maps1/1(I from batt & into bus) -> switch2/1

== system BugE_v0_40_MAS_loads/Energy Storage (New Grid)/MB2 ==
  Requested power [W] : Inport
  Calculate SOC : Subsystem
  Compute current (nolimit) : Subsystem
  Constant : Constant  Value=0  SampleTime=sample_time
  Demux : Demux  Outputs=2
  Energy Quantification : Subsystem
  "Pack Voc, R" : Subsystem
  Switch : Switch  Criteria=u2 > Threshold
  Terminator : Terminator
  and : Logic  AllPortsSameDT=off  OutDataTypeStr=boolean
  prevent timing errors : UnitDelay  SampleTime=sample_time
  tag scope: SOC_MB2=global, V_MB2_sensor=global
  wires:
  "Pack Voc, R"/2(Pack R [Ohm]) -> Compute current (nolimit)/2(Rint [Ohm]), Energy Quantification/3(In1)
  "Pack Voc, R"/1(Pack Voc [V]) -> Compute current (nolimit)/1(Voc [V])
  Compute current (nolimit)/1(I [A]) -> Energy Quantification/2(In3), Calculate SOC/2(I [A])
  Calculate SOC/1(SOC) -> [SOC_MB2]
  Compute current (nolimit)/2(V [V]) -> [V_MB2_sensor], Energy Quantification/1(In2)
  Switch/1 -> "Pack Voc, R"/2(Req. power [W]), Compute current (nolimit)/3(Output power [W])
  [temp_MB2_sensor] -> "Pack Voc, R"/3(Temp [degC]), Calculate SOC/1(Temp [C])
  [SOC_MB2] -> "Pack Voc, R"/1(SOC_prev)
  Constant/1 -> Switch/3
  Requested power [W]/1 -> Switch/1
  Demux/1 -> Terminator/1
  Demux/2 -> Switch/2
  prevent timing errors/1 -> Demux/1
  [RLY_MB] -> and/1
  [MB_MOD_PWR] -> and/2
  and/1 -> prevent timing errors/1

== system BugE_v0_40_MAS_loads/Energy Storage (New Grid)/MB2 DCDC ==
  V batt : Inport
  V bus : Inport  Port=2
  "cmd type 0 P, 1 V " : Inport  Port=3
  cmd value : Inport  Port=4
  I motor : Inport  Port=5
  0 : Constant  Value=eps  SampleTime=sample_time
  Current limiter : Subsystem
  Demux : Demux  Outputs=2
  Demux1 : Demux  Outputs=2
  Demux2 : Demux  Outputs=2
  Energy Quantification : Subsystem
  Imax abs : Constant  Value=MC_Imax  SampleTime=sample_time
  Term : Terminator
  Term1 : Terminator
  V MB nominal : Constant  Value=ess_nominal_volts*ess_module_series  SampleTime=sample_time
  eff_maps : Subsystem
  eff_maps1 : Subsystem
  enabled : Switch  Criteria=u2 > Threshold
  failure mode : Switch  Criteria=u2 > Threshold
  prevent timing errors{,1..3} (4 alike) : UnitDelay  SampleTime=sample_time
  switch2 : Switch  Criteria=u2 > Threshold
  DAB_I_in : Outport
  DAB_I_out : Outport  Port=2
  tag scope: Iin_MB2_DCDC_sensor=global, Iout_MB2_DCDC_sensor=global, Vin_MB2_DCDC=global
  wires:
  Current limiter/2(I bus side lim) -> Energy Quantification/1(In1), DAB_I_out/1, [Iout_MB2_DCDC_sensor]
  Current limiter/1(I batt side lim) -> [Iin_MB2_DCDC_sensor], DAB_I_in/1, Energy Quantification/3(In3)
  V MB nominal/1 -> failure mode/3
  failure mode/1 -> enabled/1
  [RLY_MB] -> prevent timing errors3/1
  [V_MB2_sensor] -> failure mode/1
  Demux/2 -> failure mode/2
  Demux/1 -> Term/1
  Imax abs/1 -> Current limiter/4(I max)
  cmd value/1 -> prevent timing errors2/1
  V batt/1 -> eff_maps/3(Vbatt), Energy Quantification/4(In4)
  V bus/1 -> eff_maps1/3(Vbus), eff_maps/2(Vbus), Energy Quantification/2(In2)
  Demux1/1 -> Current limiter/2(I batt side raw)
  Demux1/2 -> Current limiter/3(I bus side raw)
  "cmd type 0 P, 1 V "/1 -> prevent timing errors1/1
  eff_maps/1(I from batt & into bus) -> switch2/3
  I motor/1 -> eff_maps1/1(I motor)
  switch2/1 -> Demux1/1
  [MB_MOD_PWR] -> prevent timing errors/1
  Demux2/1 -> Term1/1
  enabled/1 -> [Vin_MB2_DCDC]
  0/1 -> enabled/3
  Demux2/2 -> Current limiter/1(enable DCDC), enabled/2
  prevent timing errors/1 -> Demux2/1
  prevent timing errors3/1 -> Demux/1
  prevent timing errors2/1 -> eff_maps1/2(Vbatt cmd), eff_maps/1("P into bus cmd ")
  eff_maps1/1(I from batt & into bus) -> switch2/1
  prevent timing errors1/1 -> switch2/2

== system BugE_v0_40_MAS_loads/Energy Storage (New Grid)/PV_cells Pout ==
  Energy Quantification : Subsystem
  power : Outport
  tag scope: PV_Pout_calc=global
  wires:
  [PV_power_lim] -> Energy Quantification/1(Power), power/1, [PV_Pout_calc]

== system BugE_v0_40_MAS_loads/Energy Storage (New Grid)/SB1 ==
  Requested power [W] : Inport
  Calculate SOC : Subsystem
  Compute current (nolimit) : Subsystem
  Constant : Constant  Value=0  SampleTime=sample_time
  Demux : Demux  Outputs=2
  Energy Quantification : Subsystem
  "Pack Voc, R" : Subsystem
  Switch : Switch  Criteria=u2 > Threshold
  Terminator : Terminator
  and : Logic  AllPortsSameDT=off  OutDataTypeStr=boolean
  prevent timing errors : UnitDelay  SampleTime=sample_time
  tag scope: SOC_SB1=global, V_SB1_sensor=global
  wires:
  Switch/1 -> Compute current (nolimit)/3(Output power [W]), "Pack Voc, R"/2(Req. power [W])
  Calculate SOC/1(SOC) -> [SOC_SB1]
  "Pack Voc, R"/1(Pack Voc [V]) -> Compute current (nolimit)/1(Voc [V])
  [temp_SB1_sensor] -> "Pack Voc, R"/3(Temp [degC]), Calculate SOC/1(Temp [C])
  [SOC_SB1] -> "Pack Voc, R"/1(SOC_prev)
  "Pack Voc, R"/2(Pack R [Ohm]) -> Energy Quantification/3(In1), Compute current (nolimit)/2(Rint [Ohm])
  Compute current (nolimit)/1(I [A]) -> Energy Quantification/2(In3), Calculate SOC/2(I [A])
  Compute current (nolimit)/2(V [V]) -> Energy Quantification/1(In2), [V_SB1_sensor]
  Constant/1 -> Switch/3
  Requested power [W]/1 -> Switch/1
  Demux/1 -> Switch/2
  Demux/2 -> Terminator/1
  [RLY_SB] -> and/1
  [SB_MOD_PWR] -> and/2
  and/1 -> prevent timing errors/1
  prevent timing errors/1 -> Demux/1

== system BugE_v0_40_MAS_loads/Energy Storage (New Grid)/SB1 DCDC ==
  V batt : Inport
  V bus : Inport  Port=2
  "cmd type 0 P, 1 V " : Inport  Port=3
  cmd value : Inport  Port=4
  Current limiter : Subsystem
  Demux : Demux  Outputs=2
  Demux1 : Demux  Outputs=2
  Energy Quantification : Subsystem
  Imax abs : Constant  Value=MC_Imax  SampleTime=sample_time
  Term : Terminator
  Terminator : Terminator
  eff_maps1 : Subsystem
  enabled : Logic  AllPortsSameDT=off  OutDataTypeStr=boolean
  prevent timing errors : UnitDelay  SampleTime=sample_time
  prevent timing errors1 : UnitDelay  SampleTime=sample_time
  DAB_I_in : Outport
  DAB_I_out : Outport  Port=2
  tag scope: Iin_SB1_DCDC_sensor=global, Iout_SB1_DCDC_sensor=global
  wires:
  Current limiter/2(I bus side lim) -> Energy Quantification/1(In1), DAB_I_out/1, [Iout_SB1_DCDC_sensor]
  Current limiter/1(I batt side lim) -> [Iin_SB1_DCDC_sensor], DAB_I_in/1, Energy Quantification/3(In3)
  Imax abs/1 -> Current limiter/4(I max)
  cmd value/1 -> prevent timing errors1/1
  V batt/1 -> eff_maps1/3(Vbatt), Energy Quantification/4(In4)
  V bus/1 -> eff_maps1/2(Vbus), Energy Quantification/2(In2)
  Demux1/1 -> Current limiter/2(I batt side raw)
  Demux1/2 -> Current limiter/3(I bus side raw)
  eff_maps1/1(I from batt & into bus) -> Demux1/1
  Demux/1 -> prevent timing errors/1
  "cmd type 0 P, 1 V "/1 -> Terminator/1
  enabled/1 -> Demux/1
  Demux/2 -> Term/1
  [SB_MOD_PWR] -> enabled/2
  [RLY_SB] -> enabled/1
  prevent timing errors/1 -> Current limiter/1(enable DCDC)
  prevent timing errors1/1 -> eff_maps1/1("P into bus cmd ")
